simulink model "model_lqr_dol_stribeck"  (R2023a)
settings: Solver=ode45  StartTime=0.0  StopTime=12  FixedStep=dt  MaxStep=0.001  RelTol=1e-3
values from neighbouring files (symbols this model uses):
  cart_pos_allowed_error = 0.003    [program1.m]
  dead_zone_ctrl_ampl = 1.0    (= 1)    [program1.m]
  enableLinmodel = 1    [program1.m]
  F = lqr(A, B, Q, R)    [program1.m]
  IC = [      0.2;      pi - 0*pi/180;      0;      0  ]    [program1.m]
  IC_liniowy = IC - [0; pi; 0; 0]    [program1.m]
  pend_position_allowed_error = 1*pi/180    (= 0.0174532925199)    [program1.m]
  sat = [-12, 12]    [program1.m]
  track_len = 0.47    [program1.m]
undefined symbols (not defined in the file or in its folder): A, B, C, D, H
settings Model: Creator=Adam  LastModifiedBy=Adam
settings SolverCC: AlgebraicLoopSolver=TrustRegion
settings DataIOCC: ExternalInput=ind  LoadExternalInput=on  SignalLogging=off  DSMLogging=off  OutputSaveName=out  ReturnWorkspaceOutputsName=sout
settings OptimizationCC: SimCompilerOptimization=on  AccelVerboseBuild=on
settings DebuggingCC: AlgebraicLoopMsg=none  UnconnectedInputMsg=warning  UnconnectedOutputMsg=warning  UnconnectedLineMsg=warning
settings ModelReferenceCC: EnableRefExpFcnMdlSchedulingChecks=on
settings RTWCC: DLArmComputeVersion=19.05

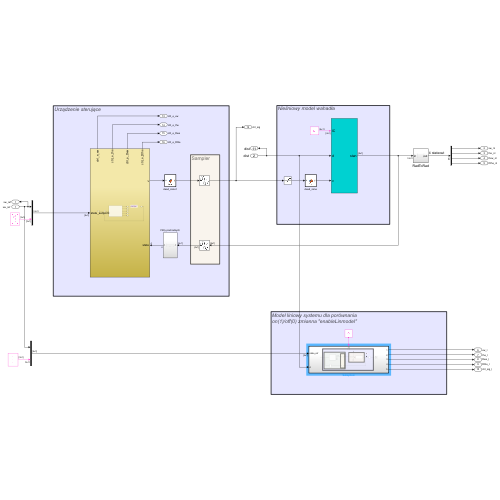
[thumbnail: Simulink's stored preview of the top-level diagram]
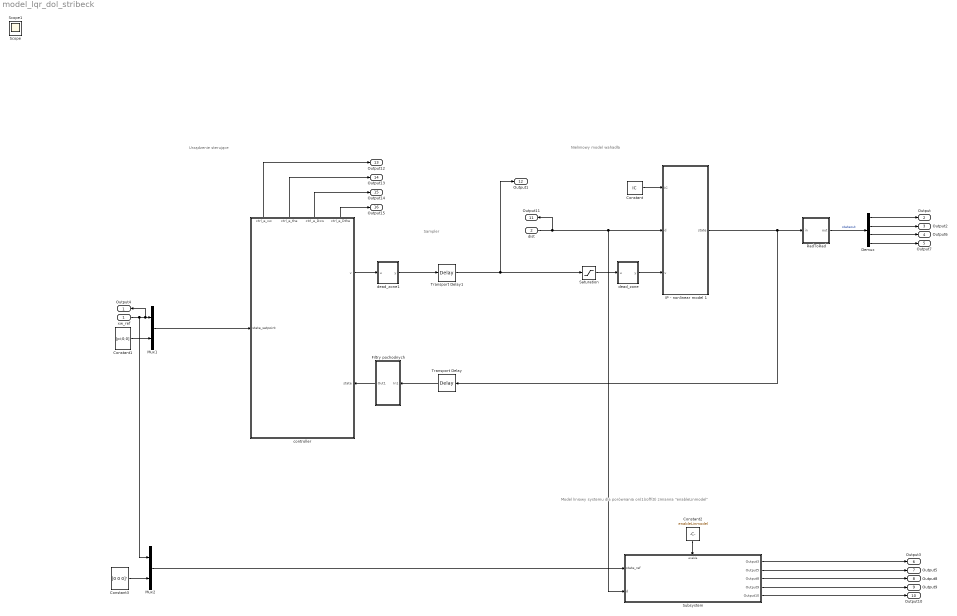
== system model_lqr_dol_stribeck ==
  note: Model liniowy systemu dla porównania
      | on(1)/off(0) zmianna "enableLinmodel"
  note: Nieliniowy model wahadła
  note: Urządzenie sterujące
  note: Sampler
  xw_ref : Inport
  dist : Inport  Port=2
  Constant : Constant  Value=IC  VectorParams1D=off
  Constant1 : Constant  Value=[pi;0;0]  VectorParams1D=off
  Constant2 : Constant  Value=enableLinmodel
  Constant3 : Constant  Value=[0 0 0]'  VectorParams1D=off
  Demux : Demux
  Filtry pochodnych : Subsystem
  IP - nonlinear model 1 : Subsystem  Description=Nonlinear model of inverted pendulum
      mask Display:
      | port_label('output', 1, 'stan');
      | port_label('input', 1, 'IC');
      | port_label('input', 2, 'd');
      | port_label('input', 3, 'v');
  Mux1 : Mux  Inputs=2
  Mux2 : Mux  Inputs=2
  RadToRad : Subsystem
  Saturation : Saturate  UpperLimit=12  LowerLimit=-12
  Subsystem : Subsystem
  Transport Delay : TransportDelay  DelayTime=0.005  InitialOutput=[track_len/2;pi;0;0]  PadeOrder=10
  Transport Delay1 : TransportDelay  DelayTime=0.005  PadeOrder=10
  controller : Subsystem
      settings: PortSchema="{\"entries\":[{\"content\":{\"sides\":[{\"content\":{\"connectorIds\":[\"In1\"]},\"type\":\"ConnectorPlacement.EquallySpacedRectSide\",\"uuid\":\"6de1dc69-5efb-4201-9eee-dce886879f47\"},{\"content\":{\"connectorIds\":[\"Out1\",\"In2\"],\"side\":\"RIGHT\"},\"type\":\"ConnectorPlacement.EquallySpacedRectSide\",\"uuid\":\"f5fecc05-d223-4a83-8c79-e750f1bc671b\"},{\"content\":{\"connectorIds\":[\"Out2\",\"Out3\",\"Out4\",\"Out5\"],\"side\":\"TOP\"},\"type\":\"ConnectorPlacement.EquallySpacedRectSide\",\"uuid\":\"1fb1d94d-6570-44f6-b110-6f3978b46153\"},{\"content\":{\"side\":\"BOTTOM\"},\"type\":\"ConnectorPlacement.EquallySpacedRectSide\",\"uuid\":\"0e2ce2e8-dcc3-40a5-a043-0a4da8b4955c\"}]},\"type\":\"ConnectorPlacement.EquallySpacedConnector\",\"uuid\":\"82464fa0-0bcf-47e2-bfa0-6457bd20ad21\"}],\"packageUris\":[\"http://schema.mathworks.com/mf0/Connector/R2020b\"],\"version\":\"1.0\"}"
  dead_zone : MATLAB Function  TreatAsAtomicUnit=on
  dead_zone1 : MATLAB Function  TreatAsAtomicUnit=on
  Output4 : Outport  SignalName=xw_ref
  Output : Outport  Port=2  SignalName=xw_nl
  Output2 : Outport  Port=3  SignalName=the_nl
  Output6 : Outport  Port=4  SignalName=Dxw_nl
  Output7 : Outport  Port=5  SignalName=Dthe_nl
  Output3 : Outport  Port=6  SignalName=xw_l
  Output5 : Outport  Port=7  SignalName=the_l
  Output8 : Outport  Port=8  SignalName=Dxw_l
  Output9 : Outport  Port=9  SignalName=Dthe_l
  Output10 : Outport  Port=10  SignalName=ctrl_sig_l
  Output11 : Outport  Port=11  SignalName=dist
  Output1 : Outport  Port=12  SignalName=ctrl_sig
  Output12 : Outport  Port=13  SignalName=ctrl_e_xw
  Output13 : Outport  Port=14  SignalName=ctrl_e_the
  Output14 : Outport  Port=15  SignalName=ctrl_e_Dxw
  Output15 : Outport  Port=16  SignalName=ctrl_e_Dthe
  Scope : Scope
  Scope1 : Scope
  wires:
  IP - nonlinear model 1/1(state) -> Transport Delay/1, RadToRad/1(in)
  Constant/1 -> IP - nonlinear model 1/1(IC)
  dist/1 -> IP - nonlinear model 1/2(d), Subsystem/2(d), Output11/1
  RadToRad/1(out) -> Demux/1  "stateout"
  Constant1/1 -> Mux1/2
  xw_ref/1 -> Output4/1, Mux1/1, Mux2/1
  Demux/1 -> Output/1
  Demux/2 -> Output2/1
  Demux/3 -> Output6/1
  Demux/4 -> Output7/1
  Subsystem/1(Output3) -> Output3/1
  Subsystem/2(Output5) -> Output5/1
  Subsystem/3(Output8) -> Output8/1
  Subsystem/4(Output9) -> Output9/1
  Subsystem/5(Output10) -> Output10/1
  Constant2/1 -> Subsystem/Enable
  Constant3/1 -> Mux2/2
  Saturation/1 -> dead_zone/1(u)
  Transport Delay1/1 -> Saturation/1, Output1/1
  Transport Delay/1 -> Filtry pochodnych/1(In1)
  Mux1/1 -> controller/1(state_setpoint)
  dead_zone/1(y) -> IP - nonlinear model 1/3(v)
  Mux2/1 -> Subsystem/1(state_ref)
  controller/2(ctrl_e_xw) -> Output12/1
  controller/3(ctrl_e_the) -> Output13/1
  controller/4(ctrl_e_Dxw) -> Output14/1
  controller/5(ctrl_e_Dthe) -> Output15/1
  controller/1(v) -> dead_zone1/1(u)
  dead_zone1/1(y) -> Transport Delay1/1
  Filtry pochodnych/1(Out1) -> controller/2(state)

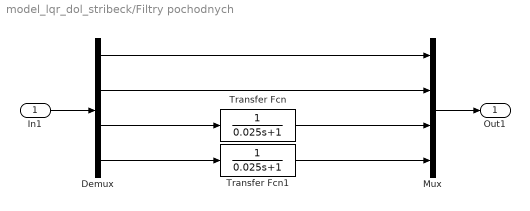
== system model_lqr_dol_stribeck/Filtry pochodnych ==
  In1 : Inport
  Demux : Demux
  Mux : Mux
  Transfer Fcn : TransferFcn  Denominator=[0.025 1]
  Transfer Fcn1 : TransferFcn  Denominator=[0.025 1]
  Out1 : Outport
  wires:
  Mux/1 -> Out1/1
  In1/1 -> Demux/1
  Demux/3 -> Transfer Fcn/1
  Demux/4 -> Transfer Fcn1/1
  Transfer Fcn1/1 -> Mux/4
  Transfer Fcn/1 -> Mux/3
  Demux/2 -> Mux/2
  Demux/1 -> Mux/1

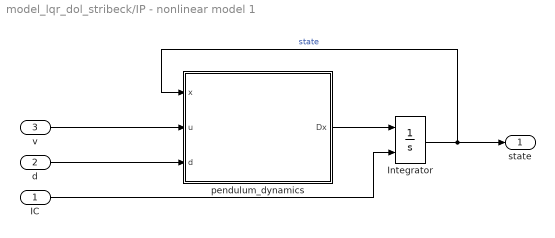
== system model_lqr_dol_stribeck/IP - nonlinear model 1 ==
  IC : Inport
  d : Inport  Port=2
  v : Inport  Port=3
  Integrator : Integrator  InitialConditionSource=external
  pendulum_dynamics : MATLAB Function  TreatAsAtomicUnit=on
  state : Outport
  wires:
  Integrator/1 -> state/1, pendulum_dynamics/1(x)  "state"
  v/1 -> pendulum_dynamics/2(u)
  pendulum_dynamics/1(Dx) -> Integrator/1
  IC/1 -> Integrator/2
  d/1 -> pendulum_dynamics/3(d)

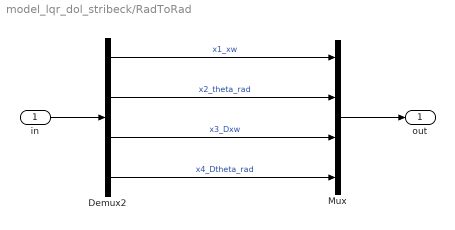
== system model_lqr_dol_stribeck/RadToRad ==
  in : Inport
  Demux2 : Demux
  Mux : Mux
  out : Outport
  wires:
  Demux2/1 -> Mux/1  "x1_xw"
  Demux2/2 -> Mux/2  "x2_theta_rad"
  in/1 -> Demux2/1
  Demux2/3 -> Mux/3  "x3_Dxw"
  Demux2/4 -> Mux/4  "x4_Dtheta_rad"
  Mux/1 -> out/1

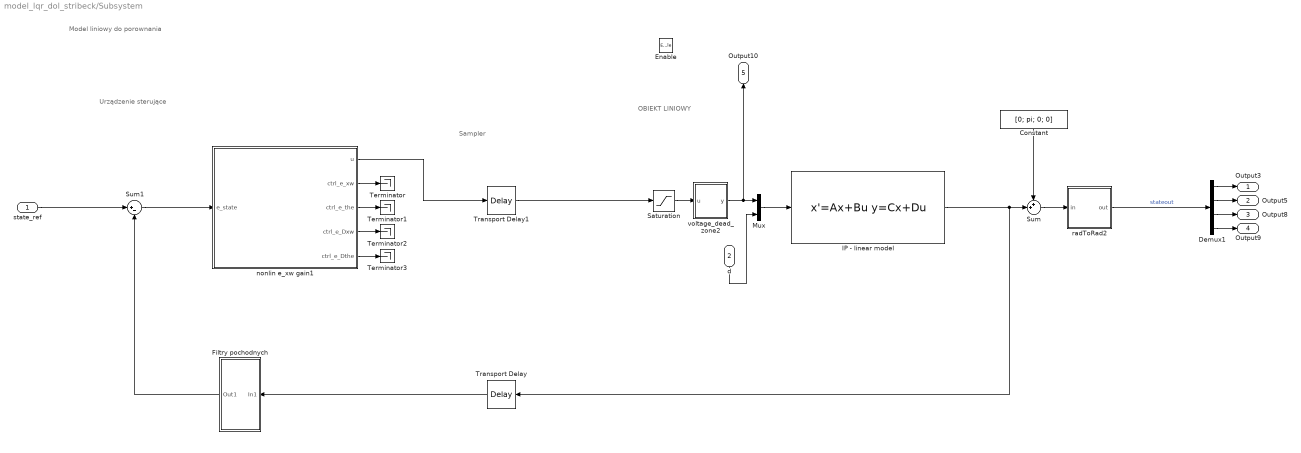
== system model_lqr_dol_stribeck/Subsystem ==
  note: OBIEKT LINIOWY
  note: Urządzenie sterujące
  note: Sampler
  note: Model liniowy do porownania
  state_ref : Inport
  d : Inport  Port=2
  Enable : EnablePort
  Constant : Constant  Value=[0; pi; 0; 0]
  Demux1 : Demux
  Filtry pochodnych : Subsystem
  IP - linear model : StateSpace  A=A  B=[B,H]  C=C  D=[D,D]  InitialCondition=IC_liniowy
  Mux : Mux  Inputs=2
  Saturation : Saturate  UpperLimit=sat(2)  LowerLimit=sat(1)
  Sum : Sum  Inputs=++|
  Sum1 : Sum  Inputs=|+-
  Terminator{,1..3} (4 alike) : Terminator
  Transport Delay : TransportDelay  DelayTime=0.005  InitialOutput=[track_len/2;0;0;0]  PadeOrder=10
  Transport Delay1 : TransportDelay  DelayTime=0.005  PadeOrder=10
  nonlin e_xw gain1 : MATLAB Function  TreatAsAtomicUnit=on
  radToRad2 : Subsystem
  voltage_dead_zone2 : MATLAB Function  TreatAsAtomicUnit=on
  Output3 : Outport
  Output5 : Outport  Port=2
  Output8 : Outport  Port=3
  Output9 : Outport  Port=4
  Output10 : Outport  Port=5
  wires:
  Transport Delay/1 -> Filtry pochodnych/1(In1)
  Transport Delay1/1 -> Saturation/1
  state_ref/1 -> Sum1/1
  Demux1/2 -> Output5/1
  Demux1/3 -> Output8/1
  Constant/1 -> Sum/1
  radToRad2/1(out) -> Demux1/1  "stateout"
  Sum/1 -> radToRad2/1(in)
  IP - linear model/1 -> Transport Delay/1, Sum/2
  Demux1/1 -> Output3/1
  Saturation/1 -> voltage_dead_zone2/1(u)
  Demux1/4 -> Output9/1
  Sum1/1 -> nonlin e_xw gain1/1(e_state)
  nonlin e_xw gain1/1(u) -> Transport Delay1/1
  nonlin e_xw gain1/2(ctrl_e_xw) -> Terminator/1
  nonlin e_xw gain1/3(ctrl_e_the) -> Terminator1/1
  nonlin e_xw gain1/4(ctrl_e_Dxw) -> Terminator2/1
  nonlin e_xw gain1/5(ctrl_e_Dthe) -> Terminator3/1
  Filtry pochodnych/1(Out1) -> Sum1/2
  Mux/1 -> IP - linear model/1
  voltage_dead_zone2/1(y) -> Output10/1, Mux/1
  d/1 -> Mux/2

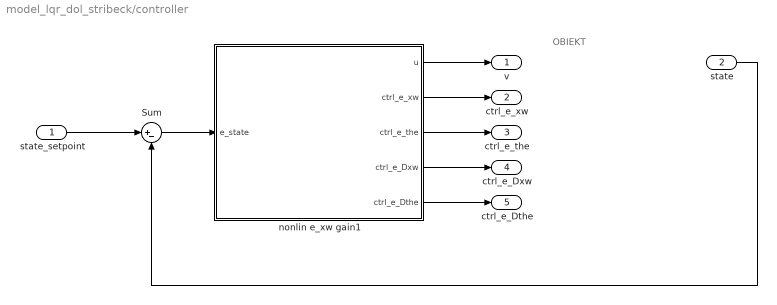
== system model_lqr_dol_stribeck/controller ==
  note: OBIEKT
  state_setpoint : Inport
  state : Inport  Port=2
  Sum : Sum  Inputs=|+-
  nonlin e_xw gain1 : MATLAB Function  TreatAsAtomicUnit=on
  v : Outport
  ctrl_e_xw : Outport  Port=2
  ctrl_e_the : Outport  Port=3
  ctrl_e_Dxw : Outport  Port=4
  ctrl_e_Dthe : Outport  Port=5
  wires:
  state_setpoint/1 -> Sum/1
  state/1 -> Sum/2
  Sum/1 -> nonlin e_xw gain1/1(e_state)
  nonlin e_xw gain1/1(u) -> v/1
  nonlin e_xw gain1/2(ctrl_e_xw) -> ctrl_e_xw/1
  nonlin e_xw gain1/3(ctrl_e_the) -> ctrl_e_the/1
  nonlin e_xw gain1/4(ctrl_e_Dxw) -> ctrl_e_Dxw/1
  nonlin e_xw gain1/5(ctrl_e_Dthe) -> ctrl_e_Dthe/1

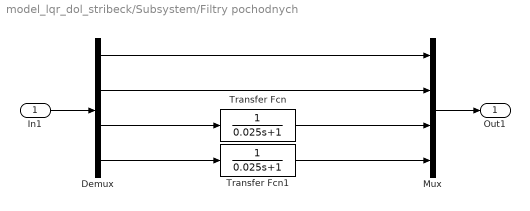
== system model_lqr_dol_stribeck/Subsystem/Filtry pochodnych ==
  In1 : Inport
  Demux : Demux
  Mux : Mux
  Transfer Fcn : TransferFcn  Denominator=[0.025 1]
  Transfer Fcn1 : TransferFcn  Denominator=[0.025 1]
  Out1 : Outport
  wires:
  Mux/1 -> Out1/1
  In1/1 -> Demux/1
  Demux/3 -> Transfer Fcn/1
  Demux/4 -> Transfer Fcn1/1
  Transfer Fcn1/1 -> Mux/4
  Transfer Fcn/1 -> Mux/3
  Demux/2 -> Mux/2
  Demux/1 -> Mux/1

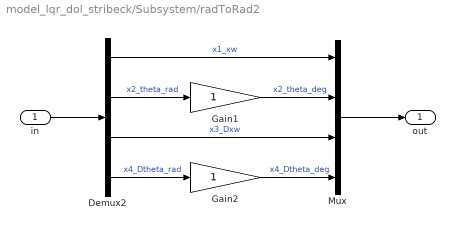
== system model_lqr_dol_stribeck/Subsystem/radToRad2 ==
  in : Inport
  Demux2 : Demux
  Gain1 : Gain
  Gain2 : Gain
  Mux : Mux
  out : Outport
  wires:
  Demux2/1 -> Mux/1  "x1_xw"
  Gain1/1 -> Mux/2  "x2_theta_deg"
  Gain2/1 -> Mux/4  "x4_Dtheta_deg"
  Demux2/2 -> Gain1/1  "x2_theta_rad"
  in/1 -> Demux2/1
  Demux2/3 -> Mux/3  "x3_Dxw"
  Demux2/4 -> Gain2/1  "x4_Dtheta_rad"
  Mux/1 -> out/1

== matlab function model_lqr_dol_stribeck/IP - nonlinear model 1/pendulum_dynamics ==
  data: x input; u input; d input; Dx output; params_nonlin_stri parameter
function Dx = dynamika_wahadla(x, u, d, params_nonlin_stri)
% x : stan
% u : input - napięcie
%
% params scope: "parameters"
%

% State, function input: x = [x Dx theta Dtheta]'
% x1 = x(1);
x2 = x(2);
x3 = x(3);
x4 = x(4);

params_stribeck = num2cell(params_nonlin_stri);
[M, mp, mc, Lp, alpha_dcm, B, gamma_stri, miu_c, miu_s, vs] = params_stribeck{:};

g = 9.8145;
Lc = 2*Lp;
mr = mc + mp;
Mt = mr + M;
L = (Lc*mc + Lp*mp) / mr;
Jcm = 1/12*mp*Lp^2;
Jt = Jcm + mr*L^2;

i_i = 2;
delta_ = 600;

Ff = (miu_c + (miu_s-miu_c)*exp(-(x3/vs)^i_i)) * Mt*g*tanh(delta_*x3);
Fi = alpha_dcm*u;
A = d*cos(x2) - Ff + L*mr*x4^2*sin(x2) - B*x3 + Fi;
B = d*Lc + L*g*mr*sin(x2) - gamma_stri*x4;
DEN = Jt*Mt - (L*mr*cos(x2))^2;

ddt_x1 = x3;
ddt_x2 = x4;
ddt_x3 = (Jt*A - L*mr*cos(x2)*B) / DEN;
ddt_x4 = (Mt*B - L*mr*cos(x2)*A) / DEN;

% output
Dx = [ddt_x1 ddt_x2 ddt_x3 ddt_x4]';

end

== matlab function model_lqr_dol_stribeck/dead_zone ==
  data: u input; y output; dead_zone_ampl parameter
function y = fcn(u, dead_zone_ampl)
    if (abs(u) < dead_zone_ampl)
        y = 0;
    else
        y = u;
    end
end

== matlab function model_lqr_dol_stribeck/Subsystem/voltage_dead_zone2 ==
  data: u input; y output; dead_zone_ampl parameter
function y = fcn(u, dead_zone_ampl)
    if (abs(u) < dead_zone_ampl)
        y = 0;
    else
        y = u;
    end
end

== matlab function model_lqr_dol_stribeck/Subsystem/nonlin e_xw gain1 ==
  data: e_state input; F parameter; u output; dead_zone_ctrl_ampl parameter; ctrl_e_xw output; ctrl_e_the output; ctrl_e_Dxw output; ctrl_e_Dthe output; cart_pos_allowed_error parameter; pend_position_allowed_error parameter
function [u, ctrl_e_xw, ctrl_e_the, ctrl_e_Dxw, ctrl_e_Dthe] = fcn(e_state, F, dead_zone_ctrl_ampl, cart_pos_allowed_error, pend_position_allowed_error)
    % ~~~~~~~~~~~~~~~~~~~~~~~~~~~~~~~~~~~~~~~~~~~~~~~~~~~~~~~~~~~~~~~~~~~~~~~~~~~~~~~~~~~~~~~~
    % Uchyby zmiennych stanu = minus zmienne przyrostowe
    % ~~~~~~~~~~~~~~~~~~~~~~~~~~~~~~~~~~~~~~~~~~~~~~~~~~~~~~~~~~~~~~~~~~~~~~~~~~~~~~~~~~~~~~~~
    e_xw     = e_state(1);
    e_the    = e_state(2);
    e_Dxw    = e_state(3);
    e_Dthe   = e_state(4);

    % % ~~~~~~~~~~~~~~~~~~~~~~~~~~~~~~~~~~~~~~~~~~~~~~~~~~~~~~~~~~~~~~~~~~~~~~~~~~~~~~~~~~~~~~~~
    % % Dozwolone błędy w położeniu wózka i wahadła - przeniesione do
    % % głównego skryptu
    % % ~~~~~~~~~~~~~~~~~~~~~~~~~~~~~~~~~~~~~~~~~~~~~~~~~~~~~~~~~~~~~~~~~~~~~~~~~~~~~~~~~~~~~~~~ 
    % cart_pos_allowed_error = 0.003;
    % pend_position_allowed_error = 1*pi/180;

    % ~~~~~~~~~~~~~~~~~~~~~~~~~~~~~~~~~~~~~~~~~~~~~~~~~~~~~~~~~~~~~~~~~~~~~~~~~~~~~~~~~~~~~~~~
    % CTRL E_XW
    % tanh na położeniu wózka
    % ~~~~~~~~~~~~~~~~~~~~~~~~~~~~~~~~~~~~~~~~~~~~~~~~~~~~~~~~~~~~~~~~~~~~~~~~~~~~~~~~~~~~~~~~
    % if( e_xw > cart_pos_allowed_error )
    %     ctrl_e_xw =   tanh( 800 * e_xw ) * ( F(1)*e_xw + dead_zone_ctrl_ampl );
    % elseif( e_xw < -cart_pos_allowed_error )
    %     ctrl_e_xw = - tanh( 800 * e_xw ) * ( F(1)*e_xw - dead_zone_ctrl_ampl );
    % else
    %     ctrl_e_xw = 0;
    % end
    if( e_xw > cart_pos_allowed_error )
        ctrl_e_xw =  F(1)*e_xw + dead_zone_ctrl_ampl;
    elseif( e_xw < -cart_pos_allowed_error )
        ctrl_e_xw =  F(1)*e_xw - dead_zone_ctrl_ampl;
    else
        ctrl_e_xw = 0;
    end
    % ctrl_e_xw = F(1)*e_xw;

    % ~~~~~~~~~~~~~~~~~~~~~~~~~~~~~~~~~~~~~~~~~~~~~~~~~~~~~~~~~~~~~~~~~~~~~~~~~~~~~~~~~~~~~~~~
    % CTRL E_THE
    % Deadzone na składowej strowania od pozycji wahadła
    % ~~~~~~~~~~~~~~~~~~~~~~~~~~~~~~~~~~~~~~~~~~~~~~~~~~~~~~~~~~~~~~~~~~~~~~~~~~~~~~~~~~~~~~~~
    if( abs( e_the ) < pend_position_allowed_error )
        ctrl_e_the = 0;
    else
        ctrl_e_the    = F(2) * e_the;
    end
    % ctrl_e_the    = F(2) * e_the;

    % ~~~~~~~~~~~~~~~~~~~~~~~~~~~~~~~~~~~~~~~~~~~~~~~~~~~~~~~~~~~~~~~~~~~~~~~~~~~~~~~~~~~~~~~~
    % CTRL E_DXW
    % ~~~~~~~~~~~~~~~~~~~~~~~~~~~~~~~~~~~~~~~~~~~~~~~~~~~~~~~~~~~~~~~~~~~~~~~~~~~~~~~~~~~~~~~~
    % if( abs( e_Dxw ) < 0.01 )
    %     ctrl_e_Dxw = 0;
    % else
    %     ctrl_e_Dxw    = Fa(3) * e_Dxw;
    % end
    ctrl_e_Dxw    = F(3) * e_Dxw;

    % ~~~~~~~~~~~~~~~~~~~~~~~~~~~~~~~~~~~~~~~~~~~~~~~~~~~~~~~~~~~~~~~~~~~~~~~~~~~~~~~~~~~~~~~~
    % CTRL E_DTHE
    % ~~~~~~~~~~~~~~~~~~~~~~~~~~~~~~~~~~~~~~~~~~~~~~~~~~~~~~~~~~~~~~~~~~~~~~~~~~~~~~~~~~~~~~~~
    ctrl_e_Dthe   = F(4) * e_Dthe;
    
    % ~~~~~~~~~~~~~~~~~~~~~~~~~~~~~~~~~~~~~~~~~~~~~~~~~~~~~~~~~~~~~~~~~~~~~~~~~~~~~~~~~~~~~~~~
    % Sygnał sterujący
    % ~~~~~~~~~~~~~~~~~~~~~~~~~~~~~~~~~~~~~~~~~~~~~~~~~~~~~~~~~~~~~~~~~~~~~~~~~~~~~~~~~~~~~~~~
    u = ctrl_e_xw + ctrl_e_the + ctrl_e_Dxw + ctrl_e_Dthe;
end

== matlab function model_lqr_dol_stribeck/controller/nonlin e_xw gain1 ==
  data: e_state input; F parameter; u output; dead_zone_ctrl_ampl parameter; ctrl_e_xw output; ctrl_e_the output; ctrl_e_Dxw output; ctrl_e_Dthe output; cart_pos_allowed_error parameter; pend_position_allowed_error parameter
function [u, ctrl_e_xw, ctrl_e_the, ctrl_e_Dxw, ctrl_e_Dthe] = fcn(e_state, F, dead_zone_ctrl_ampl, cart_pos_allowed_error, pend_position_allowed_error)
    % ~~~~~~~~~~~~~~~~~~~~~~~~~~~~~~~~~~~~~~~~~~~~~~~~~~~~~~~~~~~~~~~~~~~~~~~~~~~~~~~~~~~~~~~~
    % Uchyby zmiennych stanu = minus zmienne przyrostowe
    % ~~~~~~~~~~~~~~~~~~~~~~~~~~~~~~~~~~~~~~~~~~~~~~~~~~~~~~~~~~~~~~~~~~~~~~~~~~~~~~~~~~~~~~~~
    e_xw     = e_state(1);
    e_the    = e_state(2);
    e_Dxw    = e_state(3);
    e_Dthe   = e_state(4);

    % % ~~~~~~~~~~~~~~~~~~~~~~~~~~~~~~~~~~~~~~~~~~~~~~~~~~~~~~~~~~~~~~~~~~~~~~~~~~~~~~~~~~~~~~~~
    % % Dozwolone błędy w położeniu wózka i wahadła - przeniesione do
    % % głównego skryptu
    % % ~~~~~~~~~~~~~~~~~~~~~~~~~~~~~~~~~~~~~~~~~~~~~~~~~~~~~~~~~~~~~~~~~~~~~~~~~~~~~~~~~~~~~~~~ 
    % cart_pos_allowed_error = 0.003;
    % pend_position_allowed_error = 1*pi/180;

    % ~~~~~~~~~~~~~~~~~~~~~~~~~~~~~~~~~~~~~~~~~~~~~~~~~~~~~~~~~~~~~~~~~~~~~~~~~~~~~~~~~~~~~~~~
    % CTRL E_XW
    % tanh na położeniu wózka
    % ~~~~~~~~~~~~~~~~~~~~~~~~~~~~~~~~~~~~~~~~~~~~~~~~~~~~~~~~~~~~~~~~~~~~~~~~~~~~~~~~~~~~~~~~
    % if( e_xw > cart_pos_allowed_error )
    %     ctrl_e_xw =   tanh( 800 * e_xw ) * ( F(1)*e_xw + dead_zone_ctrl_ampl );
    % elseif( e_xw < -cart_pos_allowed_error )
    %     ctrl_e_xw = - tanh( 800 * e_xw ) * ( F(1)*e_xw - dead_zone_ctrl_ampl );
    % else
    %     ctrl_e_xw = 0;
    % end
    if( e_xw > cart_pos_allowed_error )
        ctrl_e_xw =  F(1)*e_xw + dead_zone_ctrl_ampl;
    elseif( e_xw < -cart_pos_allowed_error )
        ctrl_e_xw =  F(1)*e_xw - dead_zone_ctrl_ampl;
    else
        ctrl_e_xw = 0;
    end
    % ctrl_e_xw = F(1)*e_xw;

    % ~~~~~~~~~~~~~~~~~~~~~~~~~~~~~~~~~~~~~~~~~~~~~~~~~~~~~~~~~~~~~~~~~~~~~~~~~~~~~~~~~~~~~~~~
    % CTRL E_THE
    % Deadzone na składowej strowania od pozycji wahadła
    % ~~~~~~~~~~~~~~~~~~~~~~~~~~~~~~~~~~~~~~~~~~~~~~~~~~~~~~~~~~~~~~~~~~~~~~~~~~~~~~~~~~~~~~~~
    if( abs( e_the ) < pend_position_allowed_error )
        ctrl_e_the = 0;
    else
        ctrl_e_the    = F(2) * e_the;
    end
    % ctrl_e_the    = F(2) * e_the;

    % ~~~~~~~~~~~~~~~~~~~~~~~~~~~~~~~~~~~~~~~~~~~~~~~~~~~~~~~~~~~~~~~~~~~~~~~~~~~~~~~~~~~~~~~~
    % CTRL E_DXW
    % ~~~~~~~~~~~~~~~~~~~~~~~~~~~~~~~~~~~~~~~~~~~~~~~~~~~~~~~~~~~~~~~~~~~~~~~~~~~~~~~~~~~~~~~~
    % if( abs( e_Dxw ) < 0.01 )
    %     ctrl_e_Dxw = 0;
    % else
    %     ctrl_e_Dxw    = Fa(3) * e_Dxw;
    % end
    ctrl_e_Dxw    = F(3) * e_Dxw;

    % ~~~~~~~~~~~~~~~~~~~~~~~~~~~~~~~~~~~~~~~~~~~~~~~~~~~~~~~~~~~~~~~~~~~~~~~~~~~~~~~~~~~~~~~~
    % CTRL E_DTHE
    % ~~~~~~~~~~~~~~~~~~~~~~~~~~~~~~~~~~~~~~~~~~~~~~~~~~~~~~~~~~~~~~~~~~~~~~~~~~~~~~~~~~~~~~~~
    ctrl_e_Dthe   = F(4) * e_Dthe;
    
    % ~~~~~~~~~~~~~~~~~~~~~~~~~~~~~~~~~~~~~~~~~~~~~~~~~~~~~~~~~~~~~~~~~~~~~~~~~~~~~~~~~~~~~~~~
    % Sygnał sterujący
    % ~~~~~~~~~~~~~~~~~~~~~~~~~~~~~~~~~~~~~~~~~~~~~~~~~~~~~~~~~~~~~~~~~~~~~~~~~~~~~~~~~~~~~~~~
    u = ctrl_e_xw + ctrl_e_the + ctrl_e_Dxw + ctrl_e_Dthe;
end

== matlab function model_lqr_dol_stribeck/dead_zone1 ==
  data: u input; y output; dead_zone_ctrl_ampl parameter
function y = fcn(u, dead_zone_ctrl_ampl)
    if (abs(u) < dead_zone_ctrl_ampl)
        y = 0;
    else
        y = u;
    end
end
